simulink model "piece"  (R2018b)
settings: Solver=VariableStepAuto  StartTime=0.0  StopTime=2000  FixedStep=0.02  RelTol=1e-3
PreLoadFcn:
  | load('piece.mat')
undefined symbols (not defined in the file or in its folder): Continuous, piece, Time
libraries: sharedschedule x15, dspsrcs4 x3, ctrlSharedLib x1
settings Model: Creator=mmm  LastModifiedBy=mmm

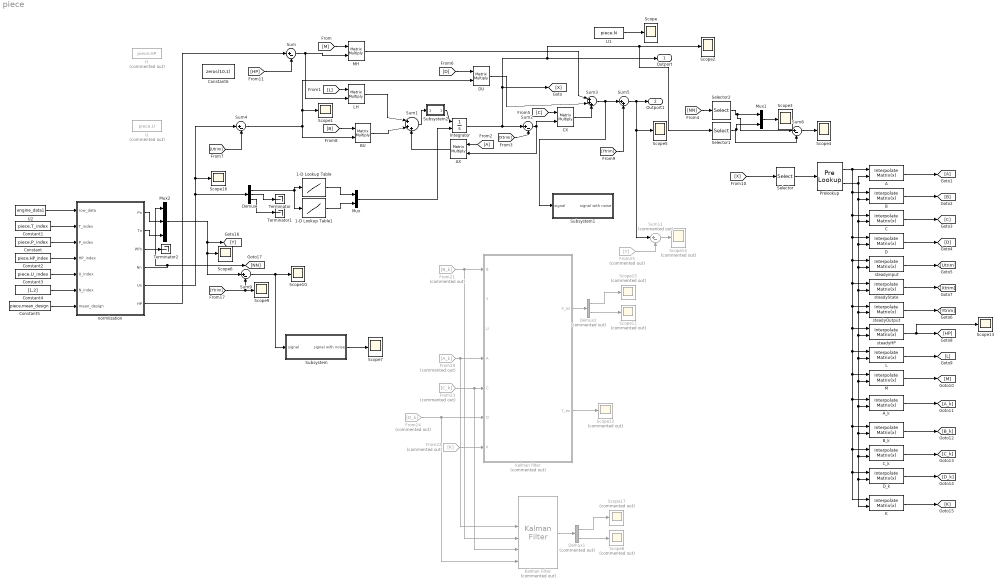
== system piece ==
  1-D Lookup Table : Lookup_n-D  NumberOfTableDimensions=1  BreakpointsForDimension1=piece.Wf_stable_(:,1)  Table=piece.Nl  InterpMethod=Cubic spline  ExtrapMethod=Cubic spline  InternalRulePriority=Speed  RndMeth=Simplest  InputSameDT=on
  1-D Lookup Table1 : Lookup_n-D  NumberOfTableDimensions=1  BreakpointsForDimension1=piece.Wf_stable_(:,1)  Table=piece.N_stable_(:,2)  InterpMethod=Cubic spline  ExtrapMethod=Cubic spline  InternalRulePriority=Speed  RndMeth=Simplest  InputSameDT=on
  A : sharedschedule/Interpolate Matrix(x)   matrix=piece.A  aMode=aMode
      settings: SourceProductName=Aerospace Blockset  SourceProductBaseCode=AE
  AX : Product  Multiplication=Matrix(*)
  A_k : sharedschedule/Interpolate Matrix(x)   matrix=piece.A_k  aMode=aMode
      settings: SourceProductName=Aerospace Blockset  SourceProductBaseCode=AE
  B : sharedschedule/Interpolate Matrix(x)   matrix=piece.B  aMode=aMode
      settings: SourceProductName=Aerospace Blockset  SourceProductBaseCode=AE
  BU : Product  Multiplication=Matrix(*)
  B_k : sharedschedule/Interpolate Matrix(x)   matrix=piece.B_k  aMode=aMode
      settings: SourceProductName=Aerospace Blockset  SourceProductBaseCode=AE
  C : sharedschedule/Interpolate Matrix(x)   matrix=piece.C  aMode=aMode
      settings: SourceProductName=Aerospace Blockset  SourceProductBaseCode=AE
  CX : Product  Multiplication=Matrix(*)
  C_k : sharedschedule/Interpolate Matrix(x)   matrix=piece.C_k  aMode=aMode
      settings: SourceProductName=Aerospace Blockset  SourceProductBaseCode=AE
  Constant : Constant  Value=piece.P_index  VectorParams1D=off
  Constant1 : Constant  Value=piece.T_index  VectorParams1D=off
  Constant2 : Constant  Value=piece.HP_index  VectorParams1D=off
  Constant3 : Constant  Value=piece.U_index  VectorParams1D=off
  Constant4 : Constant  Value=[1,2]  VectorParams1D=off
  Constant5 : Constant  Value=piece.mean_design  VectorParams1D=off
  Constant6 : Constant  Value=zeros(10,1)
  D : sharedschedule/Interpolate Matrix(x)   matrix=piece.D  aMode=aMode
      settings: SourceProductName=Aerospace Blockset  SourceProductBaseCode=AE
  DU : Product  Multiplication=Matrix(*)
  D_k : sharedschedule/Interpolate Matrix(x)   matrix=piece.D_k  aMode=aMode
      settings: SourceProductName=Aerospace Blockset  SourceProductBaseCode=AE
  Demux : Demux  Outputs=3
  Demux1 : Demux  Commented=on  Outputs=[2,10]
  Demux2 : Demux  Commented=on  Outputs=[2,10]
  From20 : From  Commented=on  GotoTag=A_k
  From21 : From  Commented=on  GotoTag=B_k
  From22 : From  Commented=on  GotoTag=K
  From23 : From  Commented=on  GotoTag=C_k
  From24 : From  Commented=on  GotoTag=D_k
  From25 : From  Commented=on  GotoTag=Y
  H : FromWorkspace  Commented=on  VariableName=piece.HP  SampleTime=0.02  Interpolate=off  OutputAfterFinalValue=Holding final value
  Integrator : Integrator  InitialConditionSource=external
  K : sharedschedule/Interpolate Matrix(x)   matrix=piece.K  aMode=aMode
      settings: SourceProductName=Aerospace Blockset  SourceProductBaseCode=AE
  Kalman Filter : ctrlSharedLib/Kalman Filter  Commented=on  TimeDomain=Continuous-Time  UseCurrentEstimator=on  ModelSource=Input port  ModelSourceVariable=ss(0.95,1,1,0,1)  A=0.95  B=1  C=1  D=0  NumberOfStates=12  NumberOfInputs=3  NumberOfOutputs=10  InitialEstimateSource=Dialog  X0=zeros(12,1)  P0=10  UseK=off  UseGH=off  NumberOfProcessNoiseInputs=1  G=1  TimeInvariantG=on  H=0  TimeInvariantH=on  Q=0.04  TimeInvariantQ=on  R=1  TimeInvariantR=on  N=0  TimeInvariantN=on  AddInputPort=on  AddEnablePort=off  OutputEstimatedY=off  OutputP=off  Ts=-1
      settings: SourceProductBaseCode=CT
  L : sharedschedule/Interpolate Matrix(x)   matrix=piece.L  aMode=aMode
      settings: SourceProductName=Aerospace Blockset  SourceProductBaseCode=AE
  LH : Product  Multiplication=Matrix(*)
  M : sharedschedule/Interpolate Matrix(x)   matrix=piece.M  aMode=aMode
      settings: SourceProductName=Aerospace Blockset  SourceProductBaseCode=AE
  MH : Product  Multiplication=Matrix(*)
  Mux : Mux  Inputs=2
  Mux1 : Mux  Inputs=2
  Mux2 : Mux  Inputs=3
  Prelookup : PreLookup  BreakpointsData=piece.Nl  BreakpointObject=Nl  ExtrapMethod=Linear  UseLastBreakpoint=on  DiagnosticForOutOfRangeInput=Warning
  Scope{,1..7,9..10,13,16} (12 alike) : Scope
  Scope{8,11..12,14..15,17} (6 alike) : Scope  Commented=on
  Selector : Selector  InputPortWidth=2  IndexOptions=Index vector (dialog)  Indices=[1]  OutputSizes=1
  Selector1 : Selector  InputPortWidth=2  IndexOptions=Index vector (dialog)  Indices=[1]  OutputSizes=1
  Selector2 : Selector  InputPortWidth=2  IndexOptions=Index vector (dialog)  Indices=[1]  OutputSizes=1
  Subsystem : Subsystem
  Subsystem1 : Subsystem
  Subsystem2 : Subsystem
  Sum{,2,4,6,9} (5 alike) : Sum  Inputs=|+-
  Sum1 : Sum  Inputs=|+++
  Sum11 : Sum  Commented=on  Inputs=|+-
  Sum3 : Sum  Inputs=|+++
  Sum5 : Sum  Inputs=|++
  Terminator : Terminator
  Terminator1 : Terminator
  Terminator2 : Terminator
  U : FromWorkspace  Commented=on  VariableName=piece.U  SampleTime=0.02  Interpolate=off  OutputAfterFinalValue=Holding final value
  U1 : FromWorkspace  VariableName=piece.N  SampleTime=0.02  Interpolate=off  OutputAfterFinalValue=Holding final value
  U2 : FromWorkspace  VariableName=engine_data1  SampleTime=0.02  Interpolate=off  OutputAfterFinalValue=Holding final value
  kalman filter : Subsystem  Commented=on
  normlization : MATLAB Function  TreatAsAtomicUnit=on
  steadyHP : sharedschedule/Interpolate Matrix(x)   matrix=piece.steadyHP  aMode=aMode
      settings: SourceProductName=Aerospace Blockset  SourceProductBaseCode=AE
  steadyOutput : sharedschedule/Interpolate Matrix(x)   matrix=piece.steadyOutput  aMode=aMode
      settings: SourceProductName=Aerospace Blockset  SourceProductBaseCode=AE
  steadyState : sharedschedule/Interpolate Matrix(x)   matrix=piece.steadyState  aMode=aMode
      settings: SourceProductName=Aerospace Blockset  SourceProductBaseCode=AE
  steadyinput : sharedschedule/Interpolate Matrix(x)   matrix=piece.steadyInput  aMode=aMode
      settings: SourceProductName=Aerospace Blockset  SourceProductBaseCode=AE
  Outport : Outport
  Outport1 : Outport  Port=2
  wires:
  [M] -> MH/1
  Sum/1 -> LH/2, MH/2
  [L] -> LH/1
  LH/1 -> Sum1/1
  BU/1 -> Sum1/2
  AX/1 -> Sum1/3
  [A] -> AX/1
  [C] -> CX/1
  CX/1 -> Sum3/3
  MH/1 -> Sum3/1
  DU/1 -> Sum3/2
  [D] -> DU/1
  Sum4/1 -> Scope1/1, DU/2, BU/2
  [B] -> BU/1
  Sum3/1 -> Subsystem1/1(signal), Sum5/1
  [Ytrim] -> Sum5/2
  Selector/1 -> Prelookup/1
  Prelookup/2 -> A/2, steadyState/2, steadyOutput/2, steadyHP/2, L/2, B_k/2, C_k/2, K/2, D_k/2, A_k/2, M/2, steadyinput/2, D/2, C/2, B/2
  Prelookup/1 -> steadyState/1, steadyOutput/1, steadyHP/1, L/1, B_k/1, C_k/1, K/1, D_k/1, A_k/1, M/1, steadyinput/1, D/1, C/1, B/1, A/1
  A/1 -> [A]
  B/1 -> [B]
  C/1 -> [C]
  D/1 -> [D]
  steadyState/1 -> [Xtrim]
  steadyOutput/1 -> [Ytrim]
  L/1 -> [L]
  steadyHP/1 -> Scope13/1, [HP]
  M/1 -> [M]
  [HP] -> Sum/2
  Demux/2 -> Terminator/1
  Demux/3 -> Terminator1/1
  Mux/1 -> Integrator/2
  Demux/1 -> 1-D Lookup Table1/1, 1-D Lookup Table/1
  1-D Lookup Table/1 -> Mux/1
  1-D Lookup Table1/1 -> Mux/2
  Sum5/1 -> Sum11/1, Scope5/1, Outport1/1
  [Utrim] -> Sum4/2
  steadyinput/1 -> [Utrim]
  [X] -> Selector/1
  Integrator/1 -> [X], Selector1/1, Scope2/1, Outport/1, Sum2/1
  Sum2/1 -> CX/2, AX/2
  [Xtrim] -> Sum2/2
  U1/1 -> Scope/1
  Mux1/1 -> Scope3/1
  Selector2/1 -> Sum6/1, Mux1/1
  Selector1/1 -> Sum6/2, Mux1/2
  Sum6/1 -> Scope4/1
  A_k/1 -> [A_k]
  D_k/1 -> [D_k]
  C_k/1 -> [C_k]
  B_k/1 -> [B_k]
  K/1 -> [K]
  Constant/1 -> normlization/3(P_index)
  Constant1/1 -> normlization/2(T_index)
  Constant2/1 -> normlization/4(HP_index)
  Constant3/1 -> normlization/5(U_index)
  Constant4/1 -> normlization/6(N_index)
  Constant5/1 -> normlization/7(mean_design)
  U2/1 -> normlization/1(row_data)
  normlization/5(Un) -> Demux/1, Scope16/1, Sum4/1
  Mux2/1 -> Scope6/1, Sum9/1, [Y]
  normlization/3(Wfn) -> Terminator2/1
  normlization/4(Nn) -> [NN], Mux2/1
  [NN] -> Selector2/1
  [Ytrim] -> Scope9/1, Sum9/2
  Sum9/1 -> Subsystem/1(signal), Scope10/1
  From22/1 -> kalman filter/7(K)
  From23/1 -> Kalman Filter/5, kalman filter/5(C)
  From21/1 -> Kalman Filter/4, kalman filter/1(B)
  From20/1 -> Kalman Filter/3, kalman filter/4(A)
  From24/1 -> Kalman Filter/6, kalman filter/6(D)
  kalman filter/1(X_es) -> Demux2/1
  Demux2/2 -> Scope11/1
  kalman filter/2(Y_es) -> Scope12/1
  From25/1 -> Sum11/2
  Sum11/1 -> Scope14/1
  Demux2/1 -> Scope15/1
  Sum1/1 -> Subsystem2/1(signal)
  Subsystem2/1(signal with noise) -> Integrator/1
  normlization/1(Pn) -> Mux2/2
  normlization/2(Tn) -> Mux2/3
  Subsystem/1(signal with noise) -> Scope7/1
  normlization/6(HP) -> Sum/1
  Demux1/1 -> Scope17/1
  Demux1/2 -> Scope8/1
  Kalman Filter/1 -> Demux1/1

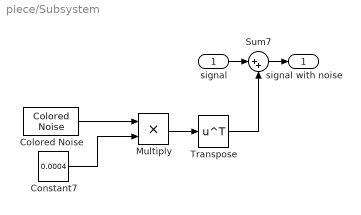
== system piece/Subsystem ==
  signal : Inport
  Colored Noise : dspsrcs4/Colored Noise  Color=white  InverseFrequencyPower=1  NumChannels=10  OutputDataType=double  SamplesPerFrame=1  SampleTime=0.02  RandomStream=mt19937ar with seed  Seed=100  SimulateUsing=Code generation
      settings: SourceProductName=DSP System Toolbox  SourceProductBaseCode=DS
  Constant7 : Constant  Value=0.0004
  Multiply : Product
  Sum7 : Sum  Inputs=|++
  Transpose : Math  Operator=transpose  SaturateOnIntegerOverflow=on
  signal with noise : Outport
  wires:
  Constant7/1 -> Multiply/2
  Colored Noise/1 -> Multiply/1
  Transpose/1 -> Sum7/2
  Multiply/1 -> Transpose/1
  signal/1 -> Sum7/1
  Sum7/1 -> signal with noise/1

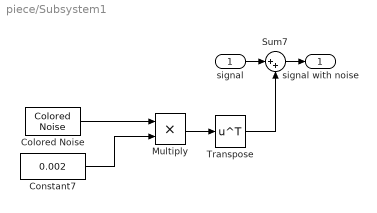
== system piece/Subsystem1 ==
  signal : Inport
  Colored Noise : dspsrcs4/Colored Noise  Color=white  InverseFrequencyPower=1  NumChannels=10  OutputDataType=double  SamplesPerFrame=1  SampleTime=0.02  RandomStream=mt19937ar with seed  Seed=100  SimulateUsing=Code generation
      settings: SourceProductName=DSP System Toolbox  SourceProductBaseCode=DS
  Constant7 : Constant  Value=0.002
  Multiply : Product
  Sum7 : Sum  Inputs=|++
  Transpose : Math  Operator=transpose  SaturateOnIntegerOverflow=on
  signal with noise : Outport
  wires:
  Sum7/1 -> signal with noise/1
  signal/1 -> Sum7/1
  Multiply/1 -> Transpose/1
  Transpose/1 -> Sum7/2
  Colored Noise/1 -> Multiply/1
  Constant7/1 -> Multiply/2

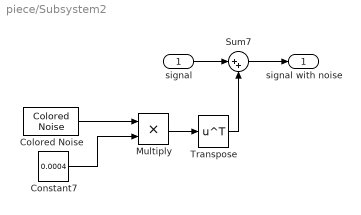
== system piece/Subsystem2 ==
  signal : Inport
  Colored Noise : dspsrcs4/Colored Noise  Color=white  InverseFrequencyPower=1  NumChannels=2  OutputDataType=double  SamplesPerFrame=1  SampleTime=0.02  RandomStream=mt19937ar with seed  Seed=222  SimulateUsing=Code generation
      settings: SourceProductName=DSP System Toolbox  SourceProductBaseCode=DS
  Constant7 : Constant  Value=0.0004
  Multiply : Product
  Sum7 : Sum  Inputs=|++
  Transpose : Math  Operator=transpose  SaturateOnIntegerOverflow=on
  signal with noise : Outport
  wires:
  Constant7/1 -> Multiply/2
  Colored Noise/1 -> Multiply/1
  Transpose/1 -> Sum7/2
  Multiply/1 -> Transpose/1
  signal/1 -> Sum7/1
  Sum7/1 -> signal with noise/1

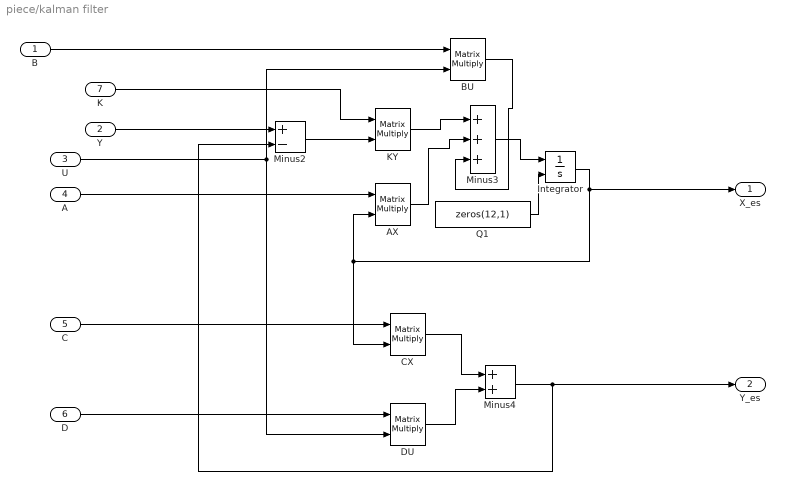
== system piece/kalman filter ==
  B : Inport
  Y : Inport  Port=2
  U : Inport  Port=3
  A : Inport  Port=4
  C : Inport  Port=5
  D : Inport  Port=6
  K : Inport  Port=7
  "\tCX" : Product  Multiplication=Matrix(*)
  AX : Product  Multiplication=Matrix(*)
  BU : Product  Multiplication=Matrix(*)
  DU : Product  Multiplication=Matrix(*)
  Integrator : Integrator  InitialConditionSource=external
  KY : Product  Multiplication=Matrix(*)
  Minus2 : Sum  Inputs=+-
  Minus3 : Sum  Inputs=+++
  Minus4 : Sum
  Q1 : Constant  Value=zeros(12,1)  VectorParams1D=off
  X_es : Outport
  Y_es : Outport  Port=2
  wires:
  Integrator/1 -> X_es/1, "\tCX"/2, AX/2
  Minus4/1 -> Minus2/2, Y_es/1
  KY/1 -> Minus3/1
  U/1 -> BU/2, DU/2
  Y/1 -> Minus2/1
  DU/1 -> Minus4/2
  AX/1 -> Minus3/2
  "\tCX"/1 -> Minus4/1
  Q1/1 -> Integrator/2
  Minus2/1 -> KY/2
  BU/1 -> Minus3/3
  Minus3/1 -> Integrator/1
  A/1 -> AX/1
  B/1 -> BU/1
  C/1 -> "\tCX"/1
  D/1 -> DU/1
  K/1 -> KY/1

== matlab function piece/normlization ==
  data: Pn output; row_data input; Tn output; T_index input; P_index input; HP_index input; U_index input; N_index input; mean_design input; Wfn output; Nn output; Un output; HP output
function [Pn,Tn,Wfn,Nn,Un,HP] = fcn(row_data,T_index,P_index,HP_index,U_index,N_index,mean_design)
%%% 数据相似归一化
if size(mean_design,1) > size(mean_design,2)
    mean_ = mean_design';
else
    mean_ = mean_design;
end
if size(T_index,1) > size(T_index,2)
    T_index_ = T_index';
else
    T_index_ = T_index;
end
if size(P_index,1) > size(P_index,2)
    P_index_ = P_index';
else
    P_index_ = P_index;
end
if size(HP_index,1) > size(HP_index,2)
    HP_index_ = HP_index';
else
    HP_index_ = HP_index;
end
if size(U_index,1) > size(U_index,2)
    U_index_ = U_index';
else
    U_index_ = U_index;
end
if size(N_index,1) > size(N_index,2)
    N_index_ = N_index';
else
    N_index_ = N_index;
end
if size(row_data,1)>size(row_data,2)
    row = row_data';
else
    row = row_data;
end
T2_index = 12;
P2_index = 13;
T = row(:,T_index_);
P = row(:,P_index_);
HP = row(:,HP_index_)'-1;
U = row(:,U_index_);
N = row(:,N_index_);
sigma_P = mean_(P_index_)./mean_(P2_index);
sigma_T = mean_(T_index_)./mean_(T2_index);
sigma_Wf = mean_(U_index_(:,1)).*sqrt(mean_(T2_index))./mean_(P2_index);
sigma_N = mean_(N_index_)./mean_(T2_index);
Tn = [(T./row(:,T2_index))./sigma_T]';
Pn = [(P./row(:,P2_index))./sigma_P]';
Wfn = (U(:,1).*sqrt(row(:,T2_index))./row(:,P2_index))./sigma_Wf;
Nn = [N./row(:,T2_index)./sigma_N]';
Un = [Wfn,U(:,2:end)]';
